simulink model "W01_Base_World_point_cloud_performance_cs"  (R2019a)
settings: Solver=FixedStepDiscrete  StartTime=0.0  StopTime=612  FixedStep=1/20  RelTol=1e-3
PreLoadFcn:
  | mbxruntime.callbacks.PreLoadFcn(bdroot);
  | check_NUTS_defined
  | model_closed = 0;
  | assignin('base',['model_closed_' bdroot],false);
PostLoadFcn:
  | mbxruntime.callbacks.PostLoadFcn(bdroot);
InitFcn:
  | mbxruntime.callbacks.InitFcn(bdroot);
StartFcn:
  | mbxruntime.callbacks.StartFcn(bdroot);
StopFcn:
  | mbxruntime.callbacks.StopFcn(bdroot);;
  | 
model workspace: external: MAT-File .\W01_Base_World_point_cloud_performance_cs_hws.mat (data not in the file)
undefined symbols (not defined in the file or in its folder): DiscIntNeverNeededParam, mbxruntime, Orientation, Position, tabledata, W01_Base_World_point_cloud_performance_cs_040d40f1a6998015, W01_Base_World_point_cloud_performance_cs_1139c7b998f0a907, W01_Base_World_point_cloud_performance_cs_282394bd9d11aaf9, W01_Base_World_point_cloud_performance_cs_287b60bdf29e1a5e, W01_Base_World_point_cloud_performance_cs_3d871abdbcb86cf3, W01_Base_World_point_cloud_performance_cs_8fcb18657fabefaa, W01_Base_World_point_cloud_performance_cs_9753c0e86959d2d1, W01_Base_World_point_cloud_performance_cs_9a36d3aa72057750, W01_Base_World_point_cloud_performance_cs_9a6e020116cabe98, W01_Base_World_point_cloud_performance_cs_a4ac4280946ec032, W01_Base_World_point_cloud_performance_cs_bbd2f0877d622aa1, W01_Base_World_point_cloud_performance_cs_d5d898f74cbe8316, W01_Base_World_point_cloud_performance_cs_d7d451946b8970f9, W01_Base_World_point_cloud_performance_cs_ed2f0fc632b9c889, W01_Base_World_point_cloud_performance_cs_f0849590441458e2, W01_Base_World_point_cloud_performance_cs_fc0d0ecba8ca3fae
libraries: simulink_extras x30, simulink x10, adeye_lib x6, sharedtransform x2, robotlib x2
(part 7 of 8)

== system W01_Base_World_point_cloud_performance_cs/TrafficLightRoadSideNL_2/Green_Mux ==
  MSCD [Cd] : Inport
  Position (xyz) [m] : Inport  Port=2
  Orientation (RPY) [deg] : Inport  Port=3
  Color [-] : Inport  Port=4
  TextureResourceID [-] : Inport  Port=5
  Bus Creator : BusCreator  Inputs='Intensity','Position','Orientation','Color','TextureResourceID'  OutDataTypeStr=Bus: PRESCAN_VISULIGHTACTUATOR_DATA  NonVirtualBus=on
  Bus Creator1 : BusCreator  Inputs=3  OutDataTypeStr=Bus: PRESCAN_RGB_DATA  NonVirtualBus=on
  Bus Creator2 : BusCreator  Inputs=3  OutDataTypeStr=Bus: PRESCAN_RPY_DATA  NonVirtualBus=on
  Bus Creator3 : BusCreator  Inputs=3  OutDataTypeStr=Bus: PRESCAN_XYZ_DATA  NonVirtualBus=on
  Data Type Conversion : DataTypeConversion  OutDataTypeStr=int32  RndMeth=Nearest
  Degrees to Radians : simulink_extras/Transformations/Degrees to Radians
  Demux : Demux  Outputs=3
  Demux1 : Demux  Outputs=3
  Demux2 : Demux  Outputs=3
  Lights : Outport
  wires:
  TextureResourceID [-]/1 -> Data Type Conversion/1  "TextureResourceID"
  MSCD [Cd]/1 -> Bus Creator/1  "Intensity"
  Bus Creator/1 -> Lights/1
  Demux/1 -> Bus Creator1/1  "R"
  Demux/2 -> Bus Creator1/2  "G"
  Demux/3 -> Bus Creator1/3  "B"
  Color [-]/1 -> Demux/1  "Color"
  Bus Creator1/1 -> Bus Creator/4  "Color"
  Demux1/1 -> Bus Creator2/1  "Roll"
  Demux1/2 -> Bus Creator2/2  "Pitch"
  Demux1/3 -> Bus Creator2/3  "Yaw"
  Orientation (RPY) [deg]/1 -> Degrees to Radians/1  "Orientation"
  Bus Creator2/1 -> Bus Creator/3  "Orientation"
  Demux2/1 -> Bus Creator3/1  "X"
  Demux2/2 -> Bus Creator3/2  "Y"
  Demux2/3 -> Bus Creator3/3  "Z"
  Position (xyz) [m]/1 -> Demux2/1  "Position"
  Bus Creator3/1 -> Bus Creator/2  "Position"
  Data Type Conversion/1 -> Bus Creator/5  "TextureResourceID"
  Degrees to Radians/1 -> Demux1/1

== system W01_Base_World_point_cloud_performance_cs/TrafficLightRoadSideNL_2/Orange_Mux ==
  MSCD [Cd] : Inport
  Position (xyz) [m] : Inport  Port=2
  Orientation (RPY) [deg] : Inport  Port=3
  Color [-] : Inport  Port=4
  TextureResourceID [-] : Inport  Port=5
  Bus Creator : BusCreator  Inputs='Intensity','Position','Orientation','Color','TextureResourceID'  OutDataTypeStr=Bus: PRESCAN_VISULIGHTACTUATOR_DATA  NonVirtualBus=on
  Bus Creator1 : BusCreator  Inputs=3  OutDataTypeStr=Bus: PRESCAN_RGB_DATA  NonVirtualBus=on
  Bus Creator2 : BusCreator  Inputs=3  OutDataTypeStr=Bus: PRESCAN_RPY_DATA  NonVirtualBus=on
  Bus Creator3 : BusCreator  Inputs=3  OutDataTypeStr=Bus: PRESCAN_XYZ_DATA  NonVirtualBus=on
  Data Type Conversion : DataTypeConversion  OutDataTypeStr=int32  RndMeth=Nearest
  Degrees to Radians : simulink_extras/Transformations/Degrees to Radians
  Demux : Demux  Outputs=3
  Demux1 : Demux  Outputs=3
  Demux2 : Demux  Outputs=3
  Lights : Outport
  wires:
  TextureResourceID [-]/1 -> Data Type Conversion/1  "TextureResourceID"
  MSCD [Cd]/1 -> Bus Creator/1  "Intensity"
  Bus Creator/1 -> Lights/1
  Demux/1 -> Bus Creator1/1  "R"
  Demux/2 -> Bus Creator1/2  "G"
  Demux/3 -> Bus Creator1/3  "B"
  Color [-]/1 -> Demux/1  "Color"
  Bus Creator1/1 -> Bus Creator/4  "Color"
  Demux1/1 -> Bus Creator2/1  "Roll"
  Demux1/2 -> Bus Creator2/2  "Pitch"
  Demux1/3 -> Bus Creator2/3  "Yaw"
  Orientation (RPY) [deg]/1 -> Degrees to Radians/1  "Orientation"
  Bus Creator2/1 -> Bus Creator/3  "Orientation"
  Demux2/1 -> Bus Creator3/1  "X"
  Demux2/2 -> Bus Creator3/2  "Y"
  Demux2/3 -> Bus Creator3/3  "Z"
  Position (xyz) [m]/1 -> Demux2/1  "Position"
  Bus Creator3/1 -> Bus Creator/2  "Position"
  Data Type Conversion/1 -> Bus Creator/5  "TextureResourceID"
  Degrees to Radians/1 -> Demux1/1

== system W01_Base_World_point_cloud_performance_cs/TrafficLightRoadSideNL_2/Red_Mux ==
  MSCD [Cd] : Inport
  Position (xyz) [m] : Inport  Port=2
  Orientation (RPY) [deg] : Inport  Port=3
  Color [-] : Inport  Port=4
  TextureResourceID [-] : Inport  Port=5
  Bus Creator : BusCreator  Inputs='Intensity','Position','Orientation','Color','TextureResourceID'  OutDataTypeStr=Bus: PRESCAN_VISULIGHTACTUATOR_DATA  NonVirtualBus=on
  Bus Creator1 : BusCreator  Inputs=3  OutDataTypeStr=Bus: PRESCAN_RGB_DATA  NonVirtualBus=on
  Bus Creator2 : BusCreator  Inputs=3  OutDataTypeStr=Bus: PRESCAN_RPY_DATA  NonVirtualBus=on
  Bus Creator3 : BusCreator  Inputs=3  OutDataTypeStr=Bus: PRESCAN_XYZ_DATA  NonVirtualBus=on
  Data Type Conversion : DataTypeConversion  OutDataTypeStr=int32  RndMeth=Nearest
  Degrees to Radians : simulink_extras/Transformations/Degrees to Radians
  Demux : Demux  Outputs=3
  Demux1 : Demux  Outputs=3
  Demux2 : Demux  Outputs=3
  Lights : Outport
  wires:
  TextureResourceID [-]/1 -> Data Type Conversion/1  "TextureResourceID"
  MSCD [Cd]/1 -> Bus Creator/1  "Intensity"
  Bus Creator/1 -> Lights/1
  Demux/1 -> Bus Creator1/1  "R"
  Demux/2 -> Bus Creator1/2  "G"
  Demux/3 -> Bus Creator1/3  "B"
  Color [-]/1 -> Demux/1  "Color"
  Bus Creator1/1 -> Bus Creator/4  "Color"
  Demux1/1 -> Bus Creator2/1  "Roll"
  Demux1/2 -> Bus Creator2/2  "Pitch"
  Demux1/3 -> Bus Creator2/3  "Yaw"
  Orientation (RPY) [deg]/1 -> Degrees to Radians/1  "Orientation"
  Bus Creator2/1 -> Bus Creator/3  "Orientation"
  Demux2/1 -> Bus Creator3/1  "X"
  Demux2/2 -> Bus Creator3/2  "Y"
  Demux2/3 -> Bus Creator3/3  "Z"
  Position (xyz) [m]/1 -> Demux2/1  "Position"
  Bus Creator3/1 -> Bus Creator/2  "Position"
  Data Type Conversion/1 -> Bus Creator/5  "TextureResourceID"
  Degrees to Radians/1 -> Demux1/1

== system W01_Base_World_point_cloud_performance_cs/TrafficLightRoadSideNL_3/Green_Mux ==
  MSCD [Cd] : Inport
  Position (xyz) [m] : Inport  Port=2
  Orientation (RPY) [deg] : Inport  Port=3
  Color [-] : Inport  Port=4
  TextureResourceID [-] : Inport  Port=5
  Bus Creator : BusCreator  Inputs='Intensity','Position','Orientation','Color','TextureResourceID'  OutDataTypeStr=Bus: PRESCAN_VISULIGHTACTUATOR_DATA  NonVirtualBus=on
  Bus Creator1 : BusCreator  Inputs=3  OutDataTypeStr=Bus: PRESCAN_RGB_DATA  NonVirtualBus=on
  Bus Creator2 : BusCreator  Inputs=3  OutDataTypeStr=Bus: PRESCAN_RPY_DATA  NonVirtualBus=on
  Bus Creator3 : BusCreator  Inputs=3  OutDataTypeStr=Bus: PRESCAN_XYZ_DATA  NonVirtualBus=on
  Data Type Conversion : DataTypeConversion  OutDataTypeStr=int32  RndMeth=Nearest
  Degrees to Radians : simulink_extras/Transformations/Degrees to Radians
  Demux : Demux  Outputs=3
  Demux1 : Demux  Outputs=3
  Demux2 : Demux  Outputs=3
  Lights : Outport
  wires:
  TextureResourceID [-]/1 -> Data Type Conversion/1  "TextureResourceID"
  MSCD [Cd]/1 -> Bus Creator/1  "Intensity"
  Bus Creator/1 -> Lights/1
  Demux/1 -> Bus Creator1/1  "R"
  Demux/2 -> Bus Creator1/2  "G"
  Demux/3 -> Bus Creator1/3  "B"
  Color [-]/1 -> Demux/1  "Color"
  Bus Creator1/1 -> Bus Creator/4  "Color"
  Demux1/1 -> Bus Creator2/1  "Roll"
  Demux1/2 -> Bus Creator2/2  "Pitch"
  Demux1/3 -> Bus Creator2/3  "Yaw"
  Orientation (RPY) [deg]/1 -> Degrees to Radians/1  "Orientation"
  Bus Creator2/1 -> Bus Creator/3  "Orientation"
  Demux2/1 -> Bus Creator3/1  "X"
  Demux2/2 -> Bus Creator3/2  "Y"
  Demux2/3 -> Bus Creator3/3  "Z"
  Position (xyz) [m]/1 -> Demux2/1  "Position"
  Bus Creator3/1 -> Bus Creator/2  "Position"
  Data Type Conversion/1 -> Bus Creator/5  "TextureResourceID"
  Degrees to Radians/1 -> Demux1/1

== system W01_Base_World_point_cloud_performance_cs/TrafficLightRoadSideNL_3/Orange_Mux ==
  MSCD [Cd] : Inport
  Position (xyz) [m] : Inport  Port=2
  Orientation (RPY) [deg] : Inport  Port=3
  Color [-] : Inport  Port=4
  TextureResourceID [-] : Inport  Port=5
  Bus Creator : BusCreator  Inputs='Intensity','Position','Orientation','Color','TextureResourceID'  OutDataTypeStr=Bus: PRESCAN_VISULIGHTACTUATOR_DATA  NonVirtualBus=on
  Bus Creator1 : BusCreator  Inputs=3  OutDataTypeStr=Bus: PRESCAN_RGB_DATA  NonVirtualBus=on
  Bus Creator2 : BusCreator  Inputs=3  OutDataTypeStr=Bus: PRESCAN_RPY_DATA  NonVirtualBus=on
  Bus Creator3 : BusCreator  Inputs=3  OutDataTypeStr=Bus: PRESCAN_XYZ_DATA  NonVirtualBus=on
  Data Type Conversion : DataTypeConversion  OutDataTypeStr=int32  RndMeth=Nearest
  Degrees to Radians : simulink_extras/Transformations/Degrees to Radians
  Demux : Demux  Outputs=3
  Demux1 : Demux  Outputs=3
  Demux2 : Demux  Outputs=3
  Lights : Outport
  wires:
  TextureResourceID [-]/1 -> Data Type Conversion/1  "TextureResourceID"
  MSCD [Cd]/1 -> Bus Creator/1  "Intensity"
  Bus Creator/1 -> Lights/1
  Demux/1 -> Bus Creator1/1  "R"
  Demux/2 -> Bus Creator1/2  "G"
  Demux/3 -> Bus Creator1/3  "B"
  Color [-]/1 -> Demux/1  "Color"
  Bus Creator1/1 -> Bus Creator/4  "Color"
  Demux1/1 -> Bus Creator2/1  "Roll"
  Demux1/2 -> Bus Creator2/2  "Pitch"
  Demux1/3 -> Bus Creator2/3  "Yaw"
  Orientation (RPY) [deg]/1 -> Degrees to Radians/1  "Orientation"
  Bus Creator2/1 -> Bus Creator/3  "Orientation"
  Demux2/1 -> Bus Creator3/1  "X"
  Demux2/2 -> Bus Creator3/2  "Y"
  Demux2/3 -> Bus Creator3/3  "Z"
  Position (xyz) [m]/1 -> Demux2/1  "Position"
  Bus Creator3/1 -> Bus Creator/2  "Position"
  Data Type Conversion/1 -> Bus Creator/5  "TextureResourceID"
  Degrees to Radians/1 -> Demux1/1

== system W01_Base_World_point_cloud_performance_cs/TrafficLightRoadSideNL_3/Red_Mux ==
  MSCD [Cd] : Inport
  Position (xyz) [m] : Inport  Port=2
  Orientation (RPY) [deg] : Inport  Port=3
  Color [-] : Inport  Port=4
  TextureResourceID [-] : Inport  Port=5
  Bus Creator : BusCreator  Inputs='Intensity','Position','Orientation','Color','TextureResourceID'  OutDataTypeStr=Bus: PRESCAN_VISULIGHTACTUATOR_DATA  NonVirtualBus=on
  Bus Creator1 : BusCreator  Inputs=3  OutDataTypeStr=Bus: PRESCAN_RGB_DATA  NonVirtualBus=on
  Bus Creator2 : BusCreator  Inputs=3  OutDataTypeStr=Bus: PRESCAN_RPY_DATA  NonVirtualBus=on
  Bus Creator3 : BusCreator  Inputs=3  OutDataTypeStr=Bus: PRESCAN_XYZ_DATA  NonVirtualBus=on
  Data Type Conversion : DataTypeConversion  OutDataTypeStr=int32  RndMeth=Nearest
  Degrees to Radians : simulink_extras/Transformations/Degrees to Radians
  Demux : Demux  Outputs=3
  Demux1 : Demux  Outputs=3
  Demux2 : Demux  Outputs=3
  Lights : Outport
  wires:
  TextureResourceID [-]/1 -> Data Type Conversion/1  "TextureResourceID"
  MSCD [Cd]/1 -> Bus Creator/1  "Intensity"
  Bus Creator/1 -> Lights/1
  Demux/1 -> Bus Creator1/1  "R"
  Demux/2 -> Bus Creator1/2  "G"
  Demux/3 -> Bus Creator1/3  "B"
  Color [-]/1 -> Demux/1  "Color"
  Bus Creator1/1 -> Bus Creator/4  "Color"
  Demux1/1 -> Bus Creator2/1  "Roll"
  Demux1/2 -> Bus Creator2/2  "Pitch"
  Demux1/3 -> Bus Creator2/3  "Yaw"
  Orientation (RPY) [deg]/1 -> Degrees to Radians/1  "Orientation"
  Bus Creator2/1 -> Bus Creator/3  "Orientation"
  Demux2/1 -> Bus Creator3/1  "X"
  Demux2/2 -> Bus Creator3/2  "Y"
  Demux2/3 -> Bus Creator3/3  "Z"
  Position (xyz) [m]/1 -> Demux2/1  "Position"
  Bus Creator3/1 -> Bus Creator/2  "Position"
  Data Type Conversion/1 -> Bus Creator/5  "TextureResourceID"
  Degrees to Radians/1 -> Demux1/1

== system W01_Base_World_point_cloud_performance_cs/TrafficLightRoadSideNL_4/Green_Mux ==
  MSCD [Cd] : Inport
  Position (xyz) [m] : Inport  Port=2
  Orientation (RPY) [deg] : Inport  Port=3
  Color [-] : Inport  Port=4
  TextureResourceID [-] : Inport  Port=5
  Bus Creator : BusCreator  Inputs='Intensity','Position','Orientation','Color','TextureResourceID'  OutDataTypeStr=Bus: PRESCAN_VISULIGHTACTUATOR_DATA  NonVirtualBus=on
  Bus Creator1 : BusCreator  Inputs=3  OutDataTypeStr=Bus: PRESCAN_RGB_DATA  NonVirtualBus=on
  Bus Creator2 : BusCreator  Inputs=3  OutDataTypeStr=Bus: PRESCAN_RPY_DATA  NonVirtualBus=on
  Bus Creator3 : BusCreator  Inputs=3  OutDataTypeStr=Bus: PRESCAN_XYZ_DATA  NonVirtualBus=on
  Data Type Conversion : DataTypeConversion  OutDataTypeStr=int32  RndMeth=Nearest
  Degrees to Radians : simulink_extras/Transformations/Degrees to Radians
  Demux : Demux  Outputs=3
  Demux1 : Demux  Outputs=3
  Demux2 : Demux  Outputs=3
  Lights : Outport
  wires:
  TextureResourceID [-]/1 -> Data Type Conversion/1  "TextureResourceID"
  MSCD [Cd]/1 -> Bus Creator/1  "Intensity"
  Bus Creator/1 -> Lights/1
  Demux/1 -> Bus Creator1/1  "R"
  Demux/2 -> Bus Creator1/2  "G"
  Demux/3 -> Bus Creator1/3  "B"
  Color [-]/1 -> Demux/1  "Color"
  Bus Creator1/1 -> Bus Creator/4  "Color"
  Demux1/1 -> Bus Creator2/1  "Roll"
  Demux1/2 -> Bus Creator2/2  "Pitch"
  Demux1/3 -> Bus Creator2/3  "Yaw"
  Orientation (RPY) [deg]/1 -> Degrees to Radians/1  "Orientation"
  Bus Creator2/1 -> Bus Creator/3  "Orientation"
  Demux2/1 -> Bus Creator3/1  "X"
  Demux2/2 -> Bus Creator3/2  "Y"
  Demux2/3 -> Bus Creator3/3  "Z"
  Position (xyz) [m]/1 -> Demux2/1  "Position"
  Bus Creator3/1 -> Bus Creator/2  "Position"
  Data Type Conversion/1 -> Bus Creator/5  "TextureResourceID"
  Degrees to Radians/1 -> Demux1/1

== system W01_Base_World_point_cloud_performance_cs/TrafficLightRoadSideNL_4/Orange_Mux ==
  MSCD [Cd] : Inport
  Position (xyz) [m] : Inport  Port=2
  Orientation (RPY) [deg] : Inport  Port=3
  Color [-] : Inport  Port=4
  TextureResourceID [-] : Inport  Port=5
  Bus Creator : BusCreator  Inputs='Intensity','Position','Orientation','Color','TextureResourceID'  OutDataTypeStr=Bus: PRESCAN_VISULIGHTACTUATOR_DATA  NonVirtualBus=on
  Bus Creator1 : BusCreator  Inputs=3  OutDataTypeStr=Bus: PRESCAN_RGB_DATA  NonVirtualBus=on
  Bus Creator2 : BusCreator  Inputs=3  OutDataTypeStr=Bus: PRESCAN_RPY_DATA  NonVirtualBus=on
  Bus Creator3 : BusCreator  Inputs=3  OutDataTypeStr=Bus: PRESCAN_XYZ_DATA  NonVirtualBus=on
  Data Type Conversion : DataTypeConversion  OutDataTypeStr=int32  RndMeth=Nearest
  Degrees to Radians : simulink_extras/Transformations/Degrees to Radians
  Demux : Demux  Outputs=3
  Demux1 : Demux  Outputs=3
  Demux2 : Demux  Outputs=3
  Lights : Outport
  wires:
  TextureResourceID [-]/1 -> Data Type Conversion/1  "TextureResourceID"
  MSCD [Cd]/1 -> Bus Creator/1  "Intensity"
  Bus Creator/1 -> Lights/1
  Demux/1 -> Bus Creator1/1  "R"
  Demux/2 -> Bus Creator1/2  "G"
  Demux/3 -> Bus Creator1/3  "B"
  Color [-]/1 -> Demux/1  "Color"
  Bus Creator1/1 -> Bus Creator/4  "Color"
  Demux1/1 -> Bus Creator2/1  "Roll"
  Demux1/2 -> Bus Creator2/2  "Pitch"
  Demux1/3 -> Bus Creator2/3  "Yaw"
  Orientation (RPY) [deg]/1 -> Degrees to Radians/1  "Orientation"
  Bus Creator2/1 -> Bus Creator/3  "Orientation"
  Demux2/1 -> Bus Creator3/1  "X"
  Demux2/2 -> Bus Creator3/2  "Y"
  Demux2/3 -> Bus Creator3/3  "Z"
  Position (xyz) [m]/1 -> Demux2/1  "Position"
  Bus Creator3/1 -> Bus Creator/2  "Position"
  Data Type Conversion/1 -> Bus Creator/5  "TextureResourceID"
  Degrees to Radians/1 -> Demux1/1

== system W01_Base_World_point_cloud_performance_cs/TrafficLightRoadSideNL_4/Red_Mux ==
  MSCD [Cd] : Inport
  Position (xyz) [m] : Inport  Port=2
  Orientation (RPY) [deg] : Inport  Port=3
  Color [-] : Inport  Port=4
  TextureResourceID [-] : Inport  Port=5
  Bus Creator : BusCreator  Inputs='Intensity','Position','Orientation','Color','TextureResourceID'  OutDataTypeStr=Bus: PRESCAN_VISULIGHTACTUATOR_DATA  NonVirtualBus=on
  Bus Creator1 : BusCreator  Inputs=3  OutDataTypeStr=Bus: PRESCAN_RGB_DATA  NonVirtualBus=on
  Bus Creator2 : BusCreator  Inputs=3  OutDataTypeStr=Bus: PRESCAN_RPY_DATA  NonVirtualBus=on
  Bus Creator3 : BusCreator  Inputs=3  OutDataTypeStr=Bus: PRESCAN_XYZ_DATA  NonVirtualBus=on
  Data Type Conversion : DataTypeConversion  OutDataTypeStr=int32  RndMeth=Nearest
  Degrees to Radians : simulink_extras/Transformations/Degrees to Radians
  Demux : Demux  Outputs=3
  Demux1 : Demux  Outputs=3
  Demux2 : Demux  Outputs=3
  Lights : Outport
  wires:
  TextureResourceID [-]/1 -> Data Type Conversion/1  "TextureResourceID"
  MSCD [Cd]/1 -> Bus Creator/1  "Intensity"
  Bus Creator/1 -> Lights/1
  Demux/1 -> Bus Creator1/1  "R"
  Demux/2 -> Bus Creator1/2  "G"
  Demux/3 -> Bus Creator1/3  "B"
  Color [-]/1 -> Demux/1  "Color"
  Bus Creator1/1 -> Bus Creator/4  "Color"
  Demux1/1 -> Bus Creator2/1  "Roll"
  Demux1/2 -> Bus Creator2/2  "Pitch"
  Demux1/3 -> Bus Creator2/3  "Yaw"
  Orientation (RPY) [deg]/1 -> Degrees to Radians/1  "Orientation"
  Bus Creator2/1 -> Bus Creator/3  "Orientation"
  Demux2/1 -> Bus Creator3/1  "X"
  Demux2/2 -> Bus Creator3/2  "Y"
  Demux2/3 -> Bus Creator3/3  "Z"
  Position (xyz) [m]/1 -> Demux2/1  "Position"
  Bus Creator3/1 -> Bus Creator/2  "Position"
  Data Type Conversion/1 -> Bus Creator/5  "TextureResourceID"
  Degrees to Radians/1 -> Demux1/1

== system W01_Base_World_point_cloud_performance_cs/TrafficLightRoadSideNL_5/Green_Mux ==
  MSCD [Cd] : Inport
  Position (xyz) [m] : Inport  Port=2
  Orientation (RPY) [deg] : Inport  Port=3
  Color [-] : Inport  Port=4
  TextureResourceID [-] : Inport  Port=5
  Bus Creator : BusCreator  Inputs='Intensity','Position','Orientation','Color','TextureResourceID'  OutDataTypeStr=Bus: PRESCAN_VISULIGHTACTUATOR_DATA  NonVirtualBus=on
  Bus Creator1 : BusCreator  Inputs=3  OutDataTypeStr=Bus: PRESCAN_RGB_DATA  NonVirtualBus=on
  Bus Creator2 : BusCreator  Inputs=3  OutDataTypeStr=Bus: PRESCAN_RPY_DATA  NonVirtualBus=on
  Bus Creator3 : BusCreator  Inputs=3  OutDataTypeStr=Bus: PRESCAN_XYZ_DATA  NonVirtualBus=on
  Data Type Conversion : DataTypeConversion  OutDataTypeStr=int32  RndMeth=Nearest
  Degrees to Radians : simulink_extras/Transformations/Degrees to Radians
  Demux : Demux  Outputs=3
  Demux1 : Demux  Outputs=3
  Demux2 : Demux  Outputs=3
  Lights : Outport
  wires:
  TextureResourceID [-]/1 -> Data Type Conversion/1  "TextureResourceID"
  MSCD [Cd]/1 -> Bus Creator/1  "Intensity"
  Bus Creator/1 -> Lights/1
  Demux/1 -> Bus Creator1/1  "R"
  Demux/2 -> Bus Creator1/2  "G"
  Demux/3 -> Bus Creator1/3  "B"
  Color [-]/1 -> Demux/1  "Color"
  Bus Creator1/1 -> Bus Creator/4  "Color"
  Demux1/1 -> Bus Creator2/1  "Roll"
  Demux1/2 -> Bus Creator2/2  "Pitch"
  Demux1/3 -> Bus Creator2/3  "Yaw"
  Orientation (RPY) [deg]/1 -> Degrees to Radians/1  "Orientation"
  Bus Creator2/1 -> Bus Creator/3  "Orientation"
  Demux2/1 -> Bus Creator3/1  "X"
  Demux2/2 -> Bus Creator3/2  "Y"
  Demux2/3 -> Bus Creator3/3  "Z"
  Position (xyz) [m]/1 -> Demux2/1  "Position"
  Bus Creator3/1 -> Bus Creator/2  "Position"
  Data Type Conversion/1 -> Bus Creator/5  "TextureResourceID"
  Degrees to Radians/1 -> Demux1/1

== system W01_Base_World_point_cloud_performance_cs/TrafficLightRoadSideNL_5/Orange_Mux ==
  MSCD [Cd] : Inport
  Position (xyz) [m] : Inport  Port=2
  Orientation (RPY) [deg] : Inport  Port=3
  Color [-] : Inport  Port=4
  TextureResourceID [-] : Inport  Port=5
  Bus Creator : BusCreator  Inputs='Intensity','Position','Orientation','Color','TextureResourceID'  OutDataTypeStr=Bus: PRESCAN_VISULIGHTACTUATOR_DATA  NonVirtualBus=on
  Bus Creator1 : BusCreator  Inputs=3  OutDataTypeStr=Bus: PRESCAN_RGB_DATA  NonVirtualBus=on
  Bus Creator2 : BusCreator  Inputs=3  OutDataTypeStr=Bus: PRESCAN_RPY_DATA  NonVirtualBus=on
  Bus Creator3 : BusCreator  Inputs=3  OutDataTypeStr=Bus: PRESCAN_XYZ_DATA  NonVirtualBus=on
  Data Type Conversion : DataTypeConversion  OutDataTypeStr=int32  RndMeth=Nearest
  Degrees to Radians : simulink_extras/Transformations/Degrees to Radians
  Demux : Demux  Outputs=3
  Demux1 : Demux  Outputs=3
  Demux2 : Demux  Outputs=3
  Lights : Outport
  wires:
  TextureResourceID [-]/1 -> Data Type Conversion/1  "TextureResourceID"
  MSCD [Cd]/1 -> Bus Creator/1  "Intensity"
  Bus Creator/1 -> Lights/1
  Demux/1 -> Bus Creator1/1  "R"
  Demux/2 -> Bus Creator1/2  "G"
  Demux/3 -> Bus Creator1/3  "B"
  Color [-]/1 -> Demux/1  "Color"
  Bus Creator1/1 -> Bus Creator/4  "Color"
  Demux1/1 -> Bus Creator2/1  "Roll"
  Demux1/2 -> Bus Creator2/2  "Pitch"
  Demux1/3 -> Bus Creator2/3  "Yaw"
  Orientation (RPY) [deg]/1 -> Degrees to Radians/1  "Orientation"
  Bus Creator2/1 -> Bus Creator/3  "Orientation"
  Demux2/1 -> Bus Creator3/1  "X"
  Demux2/2 -> Bus Creator3/2  "Y"
  Demux2/3 -> Bus Creator3/3  "Z"
  Position (xyz) [m]/1 -> Demux2/1  "Position"
  Bus Creator3/1 -> Bus Creator/2  "Position"
  Data Type Conversion/1 -> Bus Creator/5  "TextureResourceID"
  Degrees to Radians/1 -> Demux1/1

== system W01_Base_World_point_cloud_performance_cs/TrafficLightRoadSideNL_5/Red_Mux ==
  MSCD [Cd] : Inport
  Position (xyz) [m] : Inport  Port=2
  Orientation (RPY) [deg] : Inport  Port=3
  Color [-] : Inport  Port=4
  TextureResourceID [-] : Inport  Port=5
  Bus Creator : BusCreator  Inputs='Intensity','Position','Orientation','Color','TextureResourceID'  OutDataTypeStr=Bus: PRESCAN_VISULIGHTACTUATOR_DATA  NonVirtualBus=on
  Bus Creator1 : BusCreator  Inputs=3  OutDataTypeStr=Bus: PRESCAN_RGB_DATA  NonVirtualBus=on
  Bus Creator2 : BusCreator  Inputs=3  OutDataTypeStr=Bus: PRESCAN_RPY_DATA  NonVirtualBus=on
  Bus Creator3 : BusCreator  Inputs=3  OutDataTypeStr=Bus: PRESCAN_XYZ_DATA  NonVirtualBus=on
  Data Type Conversion : DataTypeConversion  OutDataTypeStr=int32  RndMeth=Nearest
  Degrees to Radians : simulink_extras/Transformations/Degrees to Radians
  Demux : Demux  Outputs=3
  Demux1 : Demux  Outputs=3
  Demux2 : Demux  Outputs=3
  Lights : Outport
  wires:
  TextureResourceID [-]/1 -> Data Type Conversion/1  "TextureResourceID"
  MSCD [Cd]/1 -> Bus Creator/1  "Intensity"
  Bus Creator/1 -> Lights/1
  Demux/1 -> Bus Creator1/1  "R"
  Demux/2 -> Bus Creator1/2  "G"
  Demux/3 -> Bus Creator1/3  "B"
  Color [-]/1 -> Demux/1  "Color"
  Bus Creator1/1 -> Bus Creator/4  "Color"
  Demux1/1 -> Bus Creator2/1  "Roll"
  Demux1/2 -> Bus Creator2/2  "Pitch"
  Demux1/3 -> Bus Creator2/3  "Yaw"
  Orientation (RPY) [deg]/1 -> Degrees to Radians/1  "Orientation"
  Bus Creator2/1 -> Bus Creator/3  "Orientation"
  Demux2/1 -> Bus Creator3/1  "X"
  Demux2/2 -> Bus Creator3/2  "Y"
  Demux2/3 -> Bus Creator3/3  "Z"
  Position (xyz) [m]/1 -> Demux2/1  "Position"
  Bus Creator3/1 -> Bus Creator/2  "Position"
  Data Type Conversion/1 -> Bus Creator/5  "TextureResourceID"
  Degrees to Radians/1 -> Demux1/1

== system W01_Base_World_point_cloud_performance_cs/TrafficLightRoadSideNL_6/Green_Mux ==
  MSCD [Cd] : Inport
  Position (xyz) [m] : Inport  Port=2
  Orientation (RPY) [deg] : Inport  Port=3
  Color [-] : Inport  Port=4
  TextureResourceID [-] : Inport  Port=5
  Bus Creator : BusCreator  Inputs='Intensity','Position','Orientation','Color','TextureResourceID'  OutDataTypeStr=Bus: PRESCAN_VISULIGHTACTUATOR_DATA  NonVirtualBus=on
  Bus Creator1 : BusCreator  Inputs=3  OutDataTypeStr=Bus: PRESCAN_RGB_DATA  NonVirtualBus=on
  Bus Creator2 : BusCreator  Inputs=3  OutDataTypeStr=Bus: PRESCAN_RPY_DATA  NonVirtualBus=on
  Bus Creator3 : BusCreator  Inputs=3  OutDataTypeStr=Bus: PRESCAN_XYZ_DATA  NonVirtualBus=on
  Data Type Conversion : DataTypeConversion  OutDataTypeStr=int32  RndMeth=Nearest
  Degrees to Radians : simulink_extras/Transformations/Degrees to Radians
  Demux : Demux  Outputs=3
  Demux1 : Demux  Outputs=3
  Demux2 : Demux  Outputs=3
  Lights : Outport
  wires:
  TextureResourceID [-]/1 -> Data Type Conversion/1  "TextureResourceID"
  MSCD [Cd]/1 -> Bus Creator/1  "Intensity"
  Bus Creator/1 -> Lights/1
  Demux/1 -> Bus Creator1/1  "R"
  Demux/2 -> Bus Creator1/2  "G"
  Demux/3 -> Bus Creator1/3  "B"
  Color [-]/1 -> Demux/1  "Color"
  Bus Creator1/1 -> Bus Creator/4  "Color"
  Demux1/1 -> Bus Creator2/1  "Roll"
  Demux1/2 -> Bus Creator2/2  "Pitch"
  Demux1/3 -> Bus Creator2/3  "Yaw"
  Orientation (RPY) [deg]/1 -> Degrees to Radians/1  "Orientation"
  Bus Creator2/1 -> Bus Creator/3  "Orientation"
  Demux2/1 -> Bus Creator3/1  "X"
  Demux2/2 -> Bus Creator3/2  "Y"
  Demux2/3 -> Bus Creator3/3  "Z"
  Position (xyz) [m]/1 -> Demux2/1  "Position"
  Bus Creator3/1 -> Bus Creator/2  "Position"
  Data Type Conversion/1 -> Bus Creator/5  "TextureResourceID"
  Degrees to Radians/1 -> Demux1/1

== system W01_Base_World_point_cloud_performance_cs/TrafficLightRoadSideNL_6/Orange_Mux ==
  MSCD [Cd] : Inport
  Position (xyz) [m] : Inport  Port=2
  Orientation (RPY) [deg] : Inport  Port=3
  Color [-] : Inport  Port=4
  TextureResourceID [-] : Inport  Port=5
  Bus Creator : BusCreator  Inputs='Intensity','Position','Orientation','Color','TextureResourceID'  OutDataTypeStr=Bus: PRESCAN_VISULIGHTACTUATOR_DATA  NonVirtualBus=on
  Bus Creator1 : BusCreator  Inputs=3  OutDataTypeStr=Bus: PRESCAN_RGB_DATA  NonVirtualBus=on
  Bus Creator2 : BusCreator  Inputs=3  OutDataTypeStr=Bus: PRESCAN_RPY_DATA  NonVirtualBus=on
  Bus Creator3 : BusCreator  Inputs=3  OutDataTypeStr=Bus: PRESCAN_XYZ_DATA  NonVirtualBus=on
  Data Type Conversion : DataTypeConversion  OutDataTypeStr=int32  RndMeth=Nearest
  Degrees to Radians : simulink_extras/Transformations/Degrees to Radians
  Demux : Demux  Outputs=3
  Demux1 : Demux  Outputs=3
  Demux2 : Demux  Outputs=3
  Lights : Outport
  wires:
  TextureResourceID [-]/1 -> Data Type Conversion/1  "TextureResourceID"
  MSCD [Cd]/1 -> Bus Creator/1  "Intensity"
  Bus Creator/1 -> Lights/1
  Demux/1 -> Bus Creator1/1  "R"
  Demux/2 -> Bus Creator1/2  "G"
  Demux/3 -> Bus Creator1/3  "B"
  Color [-]/1 -> Demux/1  "Color"
  Bus Creator1/1 -> Bus Creator/4  "Color"
  Demux1/1 -> Bus Creator2/1  "Roll"
  Demux1/2 -> Bus Creator2/2  "Pitch"
  Demux1/3 -> Bus Creator2/3  "Yaw"
  Orientation (RPY) [deg]/1 -> Degrees to Radians/1  "Orientation"
  Bus Creator2/1 -> Bus Creator/3  "Orientation"
  Demux2/1 -> Bus Creator3/1  "X"
  Demux2/2 -> Bus Creator3/2  "Y"
  Demux2/3 -> Bus Creator3/3  "Z"
  Position (xyz) [m]/1 -> Demux2/1  "Position"
  Bus Creator3/1 -> Bus Creator/2  "Position"
  Data Type Conversion/1 -> Bus Creator/5  "TextureResourceID"
  Degrees to Radians/1 -> Demux1/1

== system W01_Base_World_point_cloud_performance_cs/TrafficLightRoadSideNL_6/Red_Mux ==
  MSCD [Cd] : Inport
  Position (xyz) [m] : Inport  Port=2
  Orientation (RPY) [deg] : Inport  Port=3
  Color [-] : Inport  Port=4
  TextureResourceID [-] : Inport  Port=5
  Bus Creator : BusCreator  Inputs='Intensity','Position','Orientation','Color','TextureResourceID'  OutDataTypeStr=Bus: PRESCAN_VISULIGHTACTUATOR_DATA  NonVirtualBus=on
  Bus Creator1 : BusCreator  Inputs=3  OutDataTypeStr=Bus: PRESCAN_RGB_DATA  NonVirtualBus=on
  Bus Creator2 : BusCreator  Inputs=3  OutDataTypeStr=Bus: PRESCAN_RPY_DATA  NonVirtualBus=on
  Bus Creator3 : BusCreator  Inputs=3  OutDataTypeStr=Bus: PRESCAN_XYZ_DATA  NonVirtualBus=on
  Data Type Conversion : DataTypeConversion  OutDataTypeStr=int32  RndMeth=Nearest
  Degrees to Radians : simulink_extras/Transformations/Degrees to Radians
  Demux : Demux  Outputs=3
  Demux1 : Demux  Outputs=3
  Demux2 : Demux  Outputs=3
  Lights : Outport
  wires:
  TextureResourceID [-]/1 -> Data Type Conversion/1  "TextureResourceID"
  MSCD [Cd]/1 -> Bus Creator/1  "Intensity"
  Bus Creator/1 -> Lights/1
  Demux/1 -> Bus Creator1/1  "R"
  Demux/2 -> Bus Creator1/2  "G"
  Demux/3 -> Bus Creator1/3  "B"
  Color [-]/1 -> Demux/1  "Color"
  Bus Creator1/1 -> Bus Creator/4  "Color"
  Demux1/1 -> Bus Creator2/1  "Roll"
  Demux1/2 -> Bus Creator2/2  "Pitch"
  Demux1/3 -> Bus Creator2/3  "Yaw"
  Orientation (RPY) [deg]/1 -> Degrees to Radians/1  "Orientation"
  Bus Creator2/1 -> Bus Creator/3  "Orientation"
  Demux2/1 -> Bus Creator3/1  "X"
  Demux2/2 -> Bus Creator3/2  "Y"
  Demux2/3 -> Bus Creator3/3  "Z"
  Position (xyz) [m]/1 -> Demux2/1  "Position"
  Bus Creator3/1 -> Bus Creator/2  "Position"
  Data Type Conversion/1 -> Bus Creator/5  "TextureResourceID"
  Degrees to Radians/1 -> Demux1/1

== system W01_Base_World_point_cloud_performance_cs/TrafficLightRoadSideNL_7/Green_Mux ==
  MSCD [Cd] : Inport
  Position (xyz) [m] : Inport  Port=2
  Orientation (RPY) [deg] : Inport  Port=3
  Color [-] : Inport  Port=4
  TextureResourceID [-] : Inport  Port=5
  Bus Creator : BusCreator  Inputs='Intensity','Position','Orientation','Color','TextureResourceID'  OutDataTypeStr=Bus: PRESCAN_VISULIGHTACTUATOR_DATA  NonVirtualBus=on
  Bus Creator1 : BusCreator  Inputs=3  OutDataTypeStr=Bus: PRESCAN_RGB_DATA  NonVirtualBus=on
  Bus Creator2 : BusCreator  Inputs=3  OutDataTypeStr=Bus: PRESCAN_RPY_DATA  NonVirtualBus=on
  Bus Creator3 : BusCreator  Inputs=3  OutDataTypeStr=Bus: PRESCAN_XYZ_DATA  NonVirtualBus=on
  Data Type Conversion : DataTypeConversion  OutDataTypeStr=int32  RndMeth=Nearest
  Degrees to Radians : simulink_extras/Transformations/Degrees to Radians
  Demux : Demux  Outputs=3
  Demux1 : Demux  Outputs=3
  Demux2 : Demux  Outputs=3
  Lights : Outport
  wires:
  TextureResourceID [-]/1 -> Data Type Conversion/1  "TextureResourceID"
  MSCD [Cd]/1 -> Bus Creator/1  "Intensity"
  Bus Creator/1 -> Lights/1
  Demux/1 -> Bus Creator1/1  "R"
  Demux/2 -> Bus Creator1/2  "G"
  Demux/3 -> Bus Creator1/3  "B"
  Color [-]/1 -> Demux/1  "Color"
  Bus Creator1/1 -> Bus Creator/4  "Color"
  Demux1/1 -> Bus Creator2/1  "Roll"
  Demux1/2 -> Bus Creator2/2  "Pitch"
  Demux1/3 -> Bus Creator2/3  "Yaw"
  Orientation (RPY) [deg]/1 -> Degrees to Radians/1  "Orientation"
  Bus Creator2/1 -> Bus Creator/3  "Orientation"
  Demux2/1 -> Bus Creator3/1  "X"
  Demux2/2 -> Bus Creator3/2  "Y"
  Demux2/3 -> Bus Creator3/3  "Z"
  Position (xyz) [m]/1 -> Demux2/1  "Position"
  Bus Creator3/1 -> Bus Creator/2  "Position"
  Data Type Conversion/1 -> Bus Creator/5  "TextureResourceID"
  Degrees to Radians/1 -> Demux1/1

== system W01_Base_World_point_cloud_performance_cs/TrafficLightRoadSideNL_7/Orange_Mux ==
  MSCD [Cd] : Inport
  Position (xyz) [m] : Inport  Port=2
  Orientation (RPY) [deg] : Inport  Port=3
  Color [-] : Inport  Port=4
  TextureResourceID [-] : Inport  Port=5
  Bus Creator : BusCreator  Inputs='Intensity','Position','Orientation','Color','TextureResourceID'  OutDataTypeStr=Bus: PRESCAN_VISULIGHTACTUATOR_DATA  NonVirtualBus=on
  Bus Creator1 : BusCreator  Inputs=3  OutDataTypeStr=Bus: PRESCAN_RGB_DATA  NonVirtualBus=on
  Bus Creator2 : BusCreator  Inputs=3  OutDataTypeStr=Bus: PRESCAN_RPY_DATA  NonVirtualBus=on
  Bus Creator3 : BusCreator  Inputs=3  OutDataTypeStr=Bus: PRESCAN_XYZ_DATA  NonVirtualBus=on
  Data Type Conversion : DataTypeConversion  OutDataTypeStr=int32  RndMeth=Nearest
  Degrees to Radians : simulink_extras/Transformations/Degrees to Radians
  Demux : Demux  Outputs=3
  Demux1 : Demux  Outputs=3
  Demux2 : Demux  Outputs=3
  Lights : Outport
  wires:
  TextureResourceID [-]/1 -> Data Type Conversion/1  "TextureResourceID"
  MSCD [Cd]/1 -> Bus Creator/1  "Intensity"
  Bus Creator/1 -> Lights/1
  Demux/1 -> Bus Creator1/1  "R"
  Demux/2 -> Bus Creator1/2  "G"
  Demux/3 -> Bus Creator1/3  "B"
  Color [-]/1 -> Demux/1  "Color"
  Bus Creator1/1 -> Bus Creator/4  "Color"
  Demux1/1 -> Bus Creator2/1  "Roll"
  Demux1/2 -> Bus Creator2/2  "Pitch"
  Demux1/3 -> Bus Creator2/3  "Yaw"
  Orientation (RPY) [deg]/1 -> Degrees to Radians/1  "Orientation"
  Bus Creator2/1 -> Bus Creator/3  "Orientation"
  Demux2/1 -> Bus Creator3/1  "X"
  Demux2/2 -> Bus Creator3/2  "Y"
  Demux2/3 -> Bus Creator3/3  "Z"
  Position (xyz) [m]/1 -> Demux2/1  "Position"
  Bus Creator3/1 -> Bus Creator/2  "Position"
  Data Type Conversion/1 -> Bus Creator/5  "TextureResourceID"
  Degrees to Radians/1 -> Demux1/1

== system W01_Base_World_point_cloud_performance_cs/TrafficLightRoadSideNL_7/Red_Mux ==
  MSCD [Cd] : Inport
  Position (xyz) [m] : Inport  Port=2
  Orientation (RPY) [deg] : Inport  Port=3
  Color [-] : Inport  Port=4
  TextureResourceID [-] : Inport  Port=5
  Bus Creator : BusCreator  Inputs='Intensity','Position','Orientation','Color','TextureResourceID'  OutDataTypeStr=Bus: PRESCAN_VISULIGHTACTUATOR_DATA  NonVirtualBus=on
  Bus Creator1 : BusCreator  Inputs=3  OutDataTypeStr=Bus: PRESCAN_RGB_DATA  NonVirtualBus=on
  Bus Creator2 : BusCreator  Inputs=3  OutDataTypeStr=Bus: PRESCAN_RPY_DATA  NonVirtualBus=on
  Bus Creator3 : BusCreator  Inputs=3  OutDataTypeStr=Bus: PRESCAN_XYZ_DATA  NonVirtualBus=on
  Data Type Conversion : DataTypeConversion  OutDataTypeStr=int32  RndMeth=Nearest
  Degrees to Radians : simulink_extras/Transformations/Degrees to Radians
  Demux : Demux  Outputs=3
  Demux1 : Demux  Outputs=3
  Demux2 : Demux  Outputs=3
  Lights : Outport
  wires:
  TextureResourceID [-]/1 -> Data Type Conversion/1  "TextureResourceID"
  MSCD [Cd]/1 -> Bus Creator/1  "Intensity"
  Bus Creator/1 -> Lights/1
  Demux/1 -> Bus Creator1/1  "R"
  Demux/2 -> Bus Creator1/2  "G"
  Demux/3 -> Bus Creator1/3  "B"
  Color [-]/1 -> Demux/1  "Color"
  Bus Creator1/1 -> Bus Creator/4  "Color"
  Demux1/1 -> Bus Creator2/1  "Roll"
  Demux1/2 -> Bus Creator2/2  "Pitch"
  Demux1/3 -> Bus Creator2/3  "Yaw"
  Orientation (RPY) [deg]/1 -> Degrees to Radians/1  "Orientation"
  Bus Creator2/1 -> Bus Creator/3  "Orientation"
  Demux2/1 -> Bus Creator3/1  "X"
  Demux2/2 -> Bus Creator3/2  "Y"
  Demux2/3 -> Bus Creator3/3  "Z"
  Position (xyz) [m]/1 -> Demux2/1  "Position"
  Bus Creator3/1 -> Bus Creator/2  "Position"
  Data Type Conversion/1 -> Bus Creator/5  "TextureResourceID"
  Degrees to Radians/1 -> Demux1/1

== system W01_Base_World_point_cloud_performance_cs/TrafficLightRoadSideNL_8/Green_Mux ==
  MSCD [Cd] : Inport
  Position (xyz) [m] : Inport  Port=2
  Orientation (RPY) [deg] : Inport  Port=3
  Color [-] : Inport  Port=4
  TextureResourceID [-] : Inport  Port=5
  Bus Creator : BusCreator  Inputs='Intensity','Position','Orientation','Color','TextureResourceID'  OutDataTypeStr=Bus: PRESCAN_VISULIGHTACTUATOR_DATA  NonVirtualBus=on
  Bus Creator1 : BusCreator  Inputs=3  OutDataTypeStr=Bus: PRESCAN_RGB_DATA  NonVirtualBus=on
  Bus Creator2 : BusCreator  Inputs=3  OutDataTypeStr=Bus: PRESCAN_RPY_DATA  NonVirtualBus=on
  Bus Creator3 : BusCreator  Inputs=3  OutDataTypeStr=Bus: PRESCAN_XYZ_DATA  NonVirtualBus=on
  Data Type Conversion : DataTypeConversion  OutDataTypeStr=int32  RndMeth=Nearest
  Degrees to Radians : simulink_extras/Transformations/Degrees to Radians
  Demux : Demux  Outputs=3
  Demux1 : Demux  Outputs=3
  Demux2 : Demux  Outputs=3
  Lights : Outport
  wires:
  TextureResourceID [-]/1 -> Data Type Conversion/1  "TextureResourceID"
  MSCD [Cd]/1 -> Bus Creator/1  "Intensity"
  Bus Creator/1 -> Lights/1
  Demux/1 -> Bus Creator1/1  "R"
  Demux/2 -> Bus Creator1/2  "G"
  Demux/3 -> Bus Creator1/3  "B"
  Color [-]/1 -> Demux/1  "Color"
  Bus Creator1/1 -> Bus Creator/4  "Color"
  Demux1/1 -> Bus Creator2/1  "Roll"
  Demux1/2 -> Bus Creator2/2  "Pitch"
  Demux1/3 -> Bus Creator2/3  "Yaw"
  Orientation (RPY) [deg]/1 -> Degrees to Radians/1  "Orientation"
  Bus Creator2/1 -> Bus Creator/3  "Orientation"
  Demux2/1 -> Bus Creator3/1  "X"
  Demux2/2 -> Bus Creator3/2  "Y"
  Demux2/3 -> Bus Creator3/3  "Z"
  Position (xyz) [m]/1 -> Demux2/1  "Position"
  Bus Creator3/1 -> Bus Creator/2  "Position"
  Data Type Conversion/1 -> Bus Creator/5  "TextureResourceID"
  Degrees to Radians/1 -> Demux1/1

== system W01_Base_World_point_cloud_performance_cs/TrafficLightRoadSideNL_8/Orange_Mux ==
  MSCD [Cd] : Inport
  Position (xyz) [m] : Inport  Port=2
  Orientation (RPY) [deg] : Inport  Port=3
  Color [-] : Inport  Port=4
  TextureResourceID [-] : Inport  Port=5
  Bus Creator : BusCreator  Inputs='Intensity','Position','Orientation','Color','TextureResourceID'  OutDataTypeStr=Bus: PRESCAN_VISULIGHTACTUATOR_DATA  NonVirtualBus=on
  Bus Creator1 : BusCreator  Inputs=3  OutDataTypeStr=Bus: PRESCAN_RGB_DATA  NonVirtualBus=on
  Bus Creator2 : BusCreator  Inputs=3  OutDataTypeStr=Bus: PRESCAN_RPY_DATA  NonVirtualBus=on
  Bus Creator3 : BusCreator  Inputs=3  OutDataTypeStr=Bus: PRESCAN_XYZ_DATA  NonVirtualBus=on
  Data Type Conversion : DataTypeConversion  OutDataTypeStr=int32  RndMeth=Nearest
  Degrees to Radians : simulink_extras/Transformations/Degrees to Radians
  Demux : Demux  Outputs=3
  Demux1 : Demux  Outputs=3
  Demux2 : Demux  Outputs=3
  Lights : Outport
  wires:
  TextureResourceID [-]/1 -> Data Type Conversion/1  "TextureResourceID"
  MSCD [Cd]/1 -> Bus Creator/1  "Intensity"
  Bus Creator/1 -> Lights/1
  Demux/1 -> Bus Creator1/1  "R"
  Demux/2 -> Bus Creator1/2  "G"
  Demux/3 -> Bus Creator1/3  "B"
  Color [-]/1 -> Demux/1  "Color"
  Bus Creator1/1 -> Bus Creator/4  "Color"
  Demux1/1 -> Bus Creator2/1  "Roll"
  Demux1/2 -> Bus Creator2/2  "Pitch"
  Demux1/3 -> Bus Creator2/3  "Yaw"
  Orientation (RPY) [deg]/1 -> Degrees to Radians/1  "Orientation"
  Bus Creator2/1 -> Bus Creator/3  "Orientation"
  Demux2/1 -> Bus Creator3/1  "X"
  Demux2/2 -> Bus Creator3/2  "Y"
  Demux2/3 -> Bus Creator3/3  "Z"
  Position (xyz) [m]/1 -> Demux2/1  "Position"
  Bus Creator3/1 -> Bus Creator/2  "Position"
  Data Type Conversion/1 -> Bus Creator/5  "TextureResourceID"
  Degrees to Radians/1 -> Demux1/1

== system W01_Base_World_point_cloud_performance_cs/TrafficLightRoadSideNL_8/Red_Mux ==
  MSCD [Cd] : Inport
  Position (xyz) [m] : Inport  Port=2
  Orientation (RPY) [deg] : Inport  Port=3
  Color [-] : Inport  Port=4
  TextureResourceID [-] : Inport  Port=5
  Bus Creator : BusCreator  Inputs='Intensity','Position','Orientation','Color','TextureResourceID'  OutDataTypeStr=Bus: PRESCAN_VISULIGHTACTUATOR_DATA  NonVirtualBus=on
  Bus Creator1 : BusCreator  Inputs=3  OutDataTypeStr=Bus: PRESCAN_RGB_DATA  NonVirtualBus=on
  Bus Creator2 : BusCreator  Inputs=3  OutDataTypeStr=Bus: PRESCAN_RPY_DATA  NonVirtualBus=on
  Bus Creator3 : BusCreator  Inputs=3  OutDataTypeStr=Bus: PRESCAN_XYZ_DATA  NonVirtualBus=on
  Data Type Conversion : DataTypeConversion  OutDataTypeStr=int32  RndMeth=Nearest
  Degrees to Radians : simulink_extras/Transformations/Degrees to Radians
  Demux : Demux  Outputs=3
  Demux1 : Demux  Outputs=3
  Demux2 : Demux  Outputs=3
  Lights : Outport
  wires:
  TextureResourceID [-]/1 -> Data Type Conversion/1  "TextureResourceID"
  MSCD [Cd]/1 -> Bus Creator/1  "Intensity"
  Bus Creator/1 -> Lights/1
  Demux/1 -> Bus Creator1/1  "R"
  Demux/2 -> Bus Creator1/2  "G"
  Demux/3 -> Bus Creator1/3  "B"
  Color [-]/1 -> Demux/1  "Color"
  Bus Creator1/1 -> Bus Creator/4  "Color"
  Demux1/1 -> Bus Creator2/1  "Roll"
  Demux1/2 -> Bus Creator2/2  "Pitch"
  Demux1/3 -> Bus Creator2/3  "Yaw"
  Orientation (RPY) [deg]/1 -> Degrees to Radians/1  "Orientation"
  Bus Creator2/1 -> Bus Creator/3  "Orientation"
  Demux2/1 -> Bus Creator3/1  "X"
  Demux2/2 -> Bus Creator3/2  "Y"
  Demux2/3 -> Bus Creator3/3  "Z"
  Position (xyz) [m]/1 -> Demux2/1  "Position"
  Bus Creator3/1 -> Bus Creator/2  "Position"
  Data Type Conversion/1 -> Bus Creator/5  "TextureResourceID"
  Degrees to Radians/1 -> Demux1/1

== system W01_Base_World_point_cloud_performance_cs/Audi_A8_Sedan_1/SELF_Demux/compas converter ==
  rotz [rad] : Inport
  cart2compas : Subsystem
  rad2deg : Gain  Gain=180/pi
  heading [deg] : Outport
  wires:
  rad2deg/1 -> cart2compas/1(Angle [deg])
  rotz [rad]/1 -> rad2deg/1
  cart2compas/1(heading [deg]) -> heading [deg]/1

== system W01_Base_World_point_cloud_performance_cs/BMW_X5_SUV_1/SELF_Demux/compas converter ==
  rotz [rad] : Inport
  cart2compas : Subsystem
  rad2deg : Gain  Gain=180/pi
  heading [deg] : Outport
  wires:
  rad2deg/1 -> cart2compas/1(Angle [deg])
  rotz [rad]/1 -> rad2deg/1
  cart2compas/1(heading [deg]) -> heading [deg]/1

== system W01_Base_World_point_cloud_performance_cs/Child_RegularAni_1/Animation/animation mode ==
  vel : Inport
  Data Type Conversion : DataTypeConversion  OutDataTypeStr=double
  Fcn : Fcn  Expr=sqrt(u(1)^2+u(2)^2+u(3)^2)
  Running : simulink/Logic and Bit Operations/Compare To Constant  relop=>=  const=MWS  OutDataTypeStr=uint8  ZeroCross=off
  Sum : Sum  Inputs=|++
  Walking : simulink/Logic and Bit Operations/Compare To Zero  relop=~=  OutDataTypeStr=uint8  ZeroCross=off
  mode : Outport
  wires:
  vel/1 -> Fcn/1
  Sum/1 -> Data Type Conversion/1
  Walking/1 -> Sum/1
  Running/1 -> Sum/2
  Fcn/1 -> Walking/1, Running/1
  Data Type Conversion/1 -> mode/1

== system W01_Base_World_point_cloud_performance_cs/Child_RegularAni_1/Animation/elapsed track ==
  vel : Inport
  Discrete-Time Integrator : DiscreteIntegrator  SampleTime=-1  ICPrevOutput=DiscIntNeverNeededParam  ICPrevScaledInput=DiscIntNeverNeededParam
  Fcn : Fcn  Expr=sqrt(u(1)^2 + u(2)^2 + u(3)^2)
  s : Outport
  wires:
  Fcn/1 -> Discrete-Time Integrator/1
  vel/1 -> Fcn/1
  Discrete-Time Integrator/1 -> s/1

== system W01_Base_World_point_cloud_performance_cs/Child_RegularAni_1/SELF_Demux/compas converter ==
  rotz [rad] : Inport
  cart2compas : Subsystem
  rad2deg : Gain  Gain=180/pi
  heading [deg] : Outport
  wires:
  rad2deg/1 -> cart2compas/1(Angle [deg])
  rotz [rad]/1 -> rad2deg/1
  cart2compas/1(heading [deg]) -> heading [deg]/1

== system W01_Base_World_point_cloud_performance_cs/Child_RegularAni_2/Animation/animation mode ==
  vel : Inport
  Data Type Conversion : DataTypeConversion  OutDataTypeStr=double
  Fcn : Fcn  Expr=sqrt(u(1)^2+u(2)^2+u(3)^2)
  Running : simulink/Logic and Bit Operations/Compare To Constant  relop=>=  const=MWS  OutDataTypeStr=uint8  ZeroCross=off
  Sum : Sum  Inputs=|++
  Walking : simulink/Logic and Bit Operations/Compare To Zero  relop=~=  OutDataTypeStr=uint8  ZeroCross=off
  mode : Outport
  wires:
  vel/1 -> Fcn/1
  Sum/1 -> Data Type Conversion/1
  Walking/1 -> Sum/1
  Running/1 -> Sum/2
  Fcn/1 -> Walking/1, Running/1
  Data Type Conversion/1 -> mode/1

== system W01_Base_World_point_cloud_performance_cs/Child_RegularAni_2/Animation/elapsed track ==
  vel : Inport
  Discrete-Time Integrator : DiscreteIntegrator  SampleTime=-1  ICPrevOutput=DiscIntNeverNeededParam  ICPrevScaledInput=DiscIntNeverNeededParam
  Fcn : Fcn  Expr=sqrt(u(1)^2 + u(2)^2 + u(3)^2)
  s : Outport
  wires:
  Fcn/1 -> Discrete-Time Integrator/1
  vel/1 -> Fcn/1
  Discrete-Time Integrator/1 -> s/1

== system W01_Base_World_point_cloud_performance_cs/Child_RegularAni_2/SELF_Demux/compas converter ==
  rotz [rad] : Inport
  cart2compas : Subsystem
  rad2deg : Gain  Gain=180/pi
  heading [deg] : Outport
  wires:
  rad2deg/1 -> cart2compas/1(Angle [deg])
  rotz [rad]/1 -> rad2deg/1
  cart2compas/1(heading [deg]) -> heading [deg]/1

== system W01_Base_World_point_cloud_performance_cs/Citroen_C3_Hatchback_1/SELF_Demux/compas converter ==
  rotz [rad] : Inport
  cart2compas : Subsystem
  rad2deg : Gain  Gain=180/pi
  heading [deg] : Outport
  wires:
  rad2deg/1 -> cart2compas/1(Angle [deg])
  rotz [rad]/1 -> rad2deg/1
  cart2compas/1(heading [deg]) -> heading [deg]/1

== system W01_Base_World_point_cloud_performance_cs/Female_RegularAni_1/Animation/animation mode ==
  vel : Inport
  Data Type Conversion : DataTypeConversion  OutDataTypeStr=double
  Fcn : Fcn  Expr=sqrt(u(1)^2+u(2)^2+u(3)^2)
  Running : simulink/Logic and Bit Operations/Compare To Constant  relop=>=  const=MWS  OutDataTypeStr=uint8  ZeroCross=off
  Sum : Sum  Inputs=|++
  Walking : simulink/Logic and Bit Operations/Compare To Zero  relop=~=  OutDataTypeStr=uint8  ZeroCross=off
  mode : Outport
  wires:
  vel/1 -> Fcn/1
  Sum/1 -> Data Type Conversion/1
  Walking/1 -> Sum/1
  Running/1 -> Sum/2
  Fcn/1 -> Walking/1, Running/1
  Data Type Conversion/1 -> mode/1

== system W01_Base_World_point_cloud_performance_cs/Female_RegularAni_1/Animation/elapsed track ==
  vel : Inport
  Discrete-Time Integrator : DiscreteIntegrator  SampleTime=-1  ICPrevOutput=DiscIntNeverNeededParam  ICPrevScaledInput=DiscIntNeverNeededParam
  Fcn : Fcn  Expr=sqrt(u(1)^2 + u(2)^2 + u(3)^2)
  s : Outport
  wires:
  Fcn/1 -> Discrete-Time Integrator/1
  vel/1 -> Fcn/1
  Discrete-Time Integrator/1 -> s/1

== system W01_Base_World_point_cloud_performance_cs/Female_RegularAni_1/SELF_Demux/compas converter ==
  rotz [rad] : Inport
  cart2compas : Subsystem
  rad2deg : Gain  Gain=180/pi
  heading [deg] : Outport
  wires:
  rad2deg/1 -> cart2compas/1(Angle [deg])
  rotz [rad]/1 -> rad2deg/1
  cart2compas/1(heading [deg]) -> heading [deg]/1

== system W01_Base_World_point_cloud_performance_cs/Male_RegularAni_1/Animation/animation mode ==
  vel : Inport
  Data Type Conversion : DataTypeConversion  OutDataTypeStr=double
  Fcn : Fcn  Expr=sqrt(u(1)^2+u(2)^2+u(3)^2)
  Running : simulink/Logic and Bit Operations/Compare To Constant  relop=>=  const=MWS  OutDataTypeStr=uint8  ZeroCross=off
  Sum : Sum  Inputs=|++
  Walking : simulink/Logic and Bit Operations/Compare To Zero  relop=~=  OutDataTypeStr=uint8  ZeroCross=off
  mode : Outport
  wires:
  vel/1 -> Fcn/1
  Sum/1 -> Data Type Conversion/1
  Walking/1 -> Sum/1
  Running/1 -> Sum/2
  Fcn/1 -> Walking/1, Running/1
  Data Type Conversion/1 -> mode/1

== system W01_Base_World_point_cloud_performance_cs/Male_RegularAni_1/Animation/elapsed track ==
  vel : Inport
  Discrete-Time Integrator : DiscreteIntegrator  SampleTime=-1  ICPrevOutput=DiscIntNeverNeededParam  ICPrevScaledInput=DiscIntNeverNeededParam
  Fcn : Fcn  Expr=sqrt(u(1)^2 + u(2)^2 + u(3)^2)
  s : Outport
  wires:
  Fcn/1 -> Discrete-Time Integrator/1
  vel/1 -> Fcn/1
  Discrete-Time Integrator/1 -> s/1

== system W01_Base_World_point_cloud_performance_cs/Male_RegularAni_1/SELF_Demux/compas converter ==
  rotz [rad] : Inport
  cart2compas : Subsystem
  rad2deg : Gain  Gain=180/pi
  heading [deg] : Outport
  wires:
  rad2deg/1 -> cart2compas/1(Angle [deg])
  rotz [rad]/1 -> rad2deg/1
  cart2compas/1(heading [deg]) -> heading [deg]/1

== system W01_Base_World_point_cloud_performance_cs/Male_RegularAni_2/Animation/animation mode ==
  vel : Inport
  Data Type Conversion : DataTypeConversion  OutDataTypeStr=double
  Fcn : Fcn  Expr=sqrt(u(1)^2+u(2)^2+u(3)^2)
  Running : simulink/Logic and Bit Operations/Compare To Constant  relop=>=  const=MWS  OutDataTypeStr=uint8  ZeroCross=off
  Sum : Sum  Inputs=|++
  Walking : simulink/Logic and Bit Operations/Compare To Zero  relop=~=  OutDataTypeStr=uint8  ZeroCross=off
  mode : Outport
  wires:
  vel/1 -> Fcn/1
  Sum/1 -> Data Type Conversion/1
  Walking/1 -> Sum/1
  Running/1 -> Sum/2
  Fcn/1 -> Walking/1, Running/1
  Data Type Conversion/1 -> mode/1

== system W01_Base_World_point_cloud_performance_cs/Male_RegularAni_2/Animation/elapsed track ==
  vel : Inport
  Discrete-Time Integrator : DiscreteIntegrator  SampleTime=-1  ICPrevOutput=DiscIntNeverNeededParam  ICPrevScaledInput=DiscIntNeverNeededParam
  Fcn : Fcn  Expr=sqrt(u(1)^2 + u(2)^2 + u(3)^2)
  s : Outport
  wires:
  Fcn/1 -> Discrete-Time Integrator/1
  vel/1 -> Fcn/1
  Discrete-Time Integrator/1 -> s/1

== system W01_Base_World_point_cloud_performance_cs/Male_RegularAni_2/SELF_Demux/compas converter ==
  rotz [rad] : Inport
  cart2compas : Subsystem
  rad2deg : Gain  Gain=180/pi
  heading [deg] : Outport
  wires:
  rad2deg/1 -> cart2compas/1(Angle [deg])
  rotz [rad]/1 -> rad2deg/1
  cart2compas/1(heading [deg]) -> heading [deg]/1

== system W01_Base_World_point_cloud_performance_cs/Audi_A8_Sedan_1/SELF_Demux/compas converter/cart2compas ==
  Angle [deg] : Inport
  Constant : Constant  Value=90
  Constant1 : Constant  Value=360
  Gain : Gain  Gain=1/360
  Gain1 : Gain  Gain=360
  Gain2 : Gain  Gain=-1
  Rounding Function : Rounding
  Sum : Sum  Inputs=|-+
  Sum1 : Sum  Inputs=-+|
  Sum2 : Sum  Inputs=++|
  heading [deg] : Outport
  wires:
  Gain/1 -> Rounding Function/1
  Rounding Function/1 -> Gain1/1
  Gain1/1 -> Sum/1
  Angle [deg]/1 -> Sum1/2
  Sum/1 -> Gain2/1
  Sum1/1 -> Gain/1, Sum/2
  Constant/1 -> Sum1/1
  Gain2/1 -> Sum2/2
  Constant1/1 -> Sum2/1
  Sum2/1 -> heading [deg]/1

== system W01_Base_World_point_cloud_performance_cs/BMW_X5_SUV_1/SELF_Demux/compas converter/cart2compas ==
  Angle [deg] : Inport
  Constant : Constant  Value=90
  Constant1 : Constant  Value=360
  Gain : Gain  Gain=1/360
  Gain1 : Gain  Gain=360
  Gain2 : Gain  Gain=-1
  Rounding Function : Rounding
  Sum : Sum  Inputs=|-+
  Sum1 : Sum  Inputs=-+|
  Sum2 : Sum  Inputs=++|
  heading [deg] : Outport
  wires:
  Gain/1 -> Rounding Function/1
  Rounding Function/1 -> Gain1/1
  Gain1/1 -> Sum/1
  Angle [deg]/1 -> Sum1/2
  Sum/1 -> Gain2/1
  Sum1/1 -> Gain/1, Sum/2
  Constant/1 -> Sum1/1
  Gain2/1 -> Sum2/2
  Constant1/1 -> Sum2/1
  Sum2/1 -> heading [deg]/1

== system W01_Base_World_point_cloud_performance_cs/Child_RegularAni_1/SELF_Demux/compas converter/cart2compas ==
  Angle [deg] : Inport
  Constant : Constant  Value=90
  Constant1 : Constant  Value=360
  Gain : Gain  Gain=1/360
  Gain1 : Gain  Gain=360
  Gain2 : Gain  Gain=-1
  Rounding Function : Rounding
  Sum : Sum  Inputs=|-+
  Sum1 : Sum  Inputs=-+|
  Sum2 : Sum  Inputs=++|
  heading [deg] : Outport
  wires:
  Gain/1 -> Rounding Function/1
  Rounding Function/1 -> Gain1/1
  Gain1/1 -> Sum/1
  Angle [deg]/1 -> Sum1/2
  Sum/1 -> Gain2/1
  Sum1/1 -> Gain/1, Sum/2
  Constant/1 -> Sum1/1
  Gain2/1 -> Sum2/2
  Constant1/1 -> Sum2/1
  Sum2/1 -> heading [deg]/1

== system W01_Base_World_point_cloud_performance_cs/Child_RegularAni_2/SELF_Demux/compas converter/cart2compas ==
  Angle [deg] : Inport
  Constant : Constant  Value=90
  Constant1 : Constant  Value=360
  Gain : Gain  Gain=1/360
  Gain1 : Gain  Gain=360
  Gain2 : Gain  Gain=-1
  Rounding Function : Rounding
  Sum : Sum  Inputs=|-+
  Sum1 : Sum  Inputs=-+|
  Sum2 : Sum  Inputs=++|
  heading [deg] : Outport
  wires:
  Gain/1 -> Rounding Function/1
  Rounding Function/1 -> Gain1/1
  Gain1/1 -> Sum/1
  Angle [deg]/1 -> Sum1/2
  Sum/1 -> Gain2/1
  Sum1/1 -> Gain/1, Sum/2
  Constant/1 -> Sum1/1
  Gain2/1 -> Sum2/2
  Constant1/1 -> Sum2/1
  Sum2/1 -> heading [deg]/1
